simulink model "matrix_operations"  (R2021a)
settings: Solver=VariableStepAuto  StartTime=0.0  StopTime=10.0  RelTol=1e-3
settings Model: Creator=Acer  LastModifiedBy=Acer

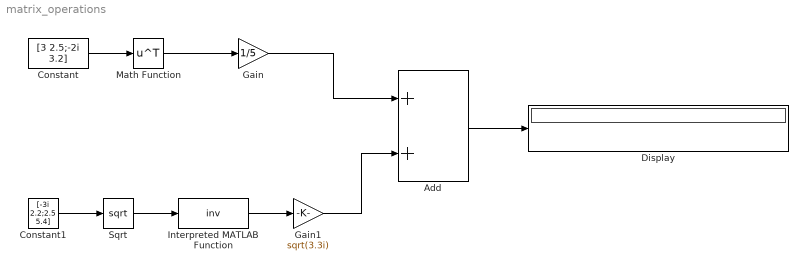
== system matrix_operations ==
  Add : Sum
  Constant : Constant  Value=[3 2.5;-2i 3.2]
  Constant1 : Constant  Value=[-3i 2.2;2.5 5.4]
  Display : Display
  Gain : Gain  Gain=1/5
  Gain1 : Gain  Gain=sqrt(3.3i)
  Interpreted MATLAB Function : MATLABFcn  MATLABFcn=inv  Output1D=off
  Math Function : Math  Operator=transpose  SaturateOnIntegerOverflow=on
  Sqrt : Sqrt  SaturateOnIntegerOverflow=on
  wires:
  Constant/1 -> Math Function/1
  Math Function/1 -> Gain/1
  Constant1/1 -> Sqrt/1
  Sqrt/1 -> Interpreted MATLAB Function/1
  Interpreted MATLAB Function/1 -> Gain1/1
  Gain/1 -> Add/1
  Gain1/1 -> Add/2
  Add/1 -> Display/1
